simulink library "ttc"  (Simulink 8.2)
settings: Solver=ode45  StartTime=0.0  StopTime=10.0  RelTol=1e-3
undefined symbols (not defined in the file or in its folder): KIFO_OffsetToBumper_m
libraries: tcc x4, idiada_lib x1
settings Model: Creator=xsellart  LastModifiedBy=14069

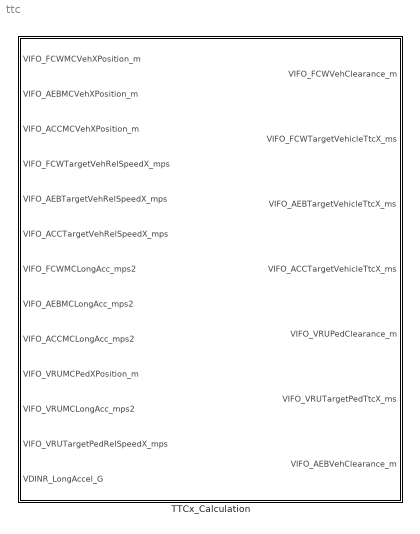
== system ttc ==
  TTCx_Calculation : Subsystem

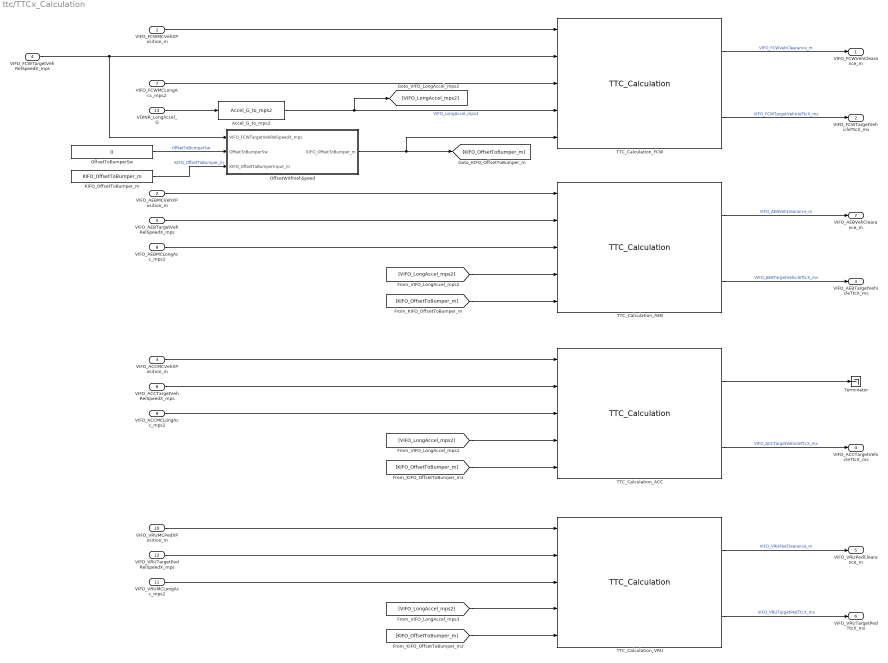
== system ttc/TTCx_Calculation ==
  VIFO_FCWMCVehXPosition_m : Inport
  VIFO_AEBMCVehXPosition_m : Inport  Port=2
  VIFO_ACCMCVehXPosition_m : Inport  Port=3
  VIFO_FCWTargetVehRelSpeedX_mps : Inport  Port=4
  VIFO_AEBTargetVehRelSpeedX_mps : Inport  Port=5
  VIFO_ACCTargetVehRelSpeedX_mps : Inport  Port=6
  VIFO_FCWMCLongAcc_mps2 : Inport  Port=7
  VIFO_AEBMCLongAcc_mps2 : Inport  Port=8
  VIFO_ACCMCLongAcc_mps2 : Inport  Port=9
  VIFO_VRUMCPedXPosition_m : Inport  Port=10
  VIFO_VRUMCLongAcc_mps2 : Inport  Port=11
  VIFO_VRUTargetPedRelSpeedX_mps : Inport  Port=12
  VDINR_LongAccel_G : Inport  Port=13
  Accel_G_to_mps2 : idiada_lib/Accel_G_to_mps2
  KIFO_OffsetToBumper_m : Constant  Value=KIFO_OffsetToBumper_m
  OffsetToBumperSw : Constant  Value=0
  OffsetWithVehSpeed : Subsystem
  TTC_Calculation_ACC : tcc/TTC_Calculation
  TTC_Calculation_AEB : tcc/TTC_Calculation
  TTC_Calculation_FCW : tcc/TTC_Calculation
  TTC_Calculation_VRU : tcc/TTC_Calculation
  Terminator : Terminator
  VIFO_FCWVehClearance_m : Outport
  VIFO_FCWTargetVehicleTtcX_ms : Outport  Port=2
  VIFO_AEBTargetVehicleTtcX_ms : Outport  Port=3
  VIFO_ACCTargetVehicleTtcX_ms : Outport  Port=4
  VIFO_VRUPedClearance_m : Outport  Port=5
  VIFO_VRUTargetPedTtcX_ms : Outport  Port=6
  VIFO_AEBVehClearance_m : Outport  Port=7
  wires:
  [KIFO_OffsetToBumper_m] -> TTC_Calculation_ACC/5
  TTC_Calculation_ACC/2 -> VIFO_ACCTargetVehicleTtcX_ms/1  "VIFO_ACCTargetVehicleTtcX_ms"
  VIFO_ACCMCLongAcc_mps2/1 -> TTC_Calculation_ACC/3
  VIFO_ACCTargetVehRelSpeedX_mps/1 -> TTC_Calculation_ACC/2
  VIFO_ACCMCVehXPosition_m/1 -> TTC_Calculation_ACC/1
  [VIFO_LongAccel_mps2] -> TTC_Calculation_ACC/4
  TTC_Calculation_ACC/1 -> Terminator/1
  [KIFO_OffsetToBumper_m] -> TTC_Calculation_AEB/5
  KIFO_OffsetToBumper_m/1 -> OffsetWithVehSpeed/3(KIFO_OffsetToBumperInput_m)  "KIFO_OffsetToBumper_m"
  TTC_Calculation_AEB/2 -> VIFO_AEBTargetVehicleTtcX_ms/1  "VIFO_AEBTargetVehicleTtcX_ms"
  VIFO_AEBMCLongAcc_mps2/1 -> TTC_Calculation_AEB/3
  VIFO_AEBTargetVehRelSpeedX_mps/1 -> TTC_Calculation_AEB/2
  VIFO_AEBMCVehXPosition_m/1 -> TTC_Calculation_AEB/1
  [VIFO_LongAccel_mps2] -> TTC_Calculation_AEB/4
  TTC_Calculation_AEB/1 -> VIFO_AEBVehClearance_m/1  "VIFO_AEBVehClearance_m"
  TTC_Calculation_FCW/2 -> VIFO_FCWTargetVehicleTtcX_ms/1  "VIFO_FCWTargetVehicleTtcX_ms"
  TTC_Calculation_FCW/1 -> VIFO_FCWVehClearance_m/1  "VIFO_FCWVehClearance_m"
  VIFO_FCWMCLongAcc_mps2/1 -> TTC_Calculation_FCW/3
  VIFO_FCWTargetVehRelSpeedX_mps/1 -> OffsetWithVehSpeed/1(VIFO_FCWTargetVehRelSpeedX_mps), TTC_Calculation_FCW/2
  VIFO_FCWMCVehXPosition_m/1 -> TTC_Calculation_FCW/1
  Accel_G_to_mps2/1 -> TTC_Calculation_FCW/4, [VIFO_LongAccel_mps2]  "VIFO_LongAccel_mps2"
  VDINR_LongAccel_G/1 -> Accel_G_to_mps2/1
  VIFO_VRUMCPedXPosition_m/1 -> TTC_Calculation_VRU/1
  VIFO_VRUTargetPedRelSpeedX_mps/1 -> TTC_Calculation_VRU/2
  VIFO_VRUMCLongAcc_mps2/1 -> TTC_Calculation_VRU/3
  [KIFO_OffsetToBumper_m] -> TTC_Calculation_VRU/5
  [VIFO_LongAccel_mps2] -> TTC_Calculation_VRU/4
  TTC_Calculation_VRU/2 -> VIFO_VRUTargetPedTtcX_ms/1  "VIFO_VRUTargetPedTtcX_ms"
  TTC_Calculation_VRU/1 -> VIFO_VRUPedClearance_m/1  "VIFO_VRUPedClearance_m"
  OffsetWithVehSpeed/1(KIFO_OffsetToBumper_m) -> TTC_Calculation_FCW/5, [KIFO_OffsetToBumper_m]
  OffsetToBumperSw/1 -> OffsetWithVehSpeed/2(OffsetToBumperSw)  "OffsetToBumperSw"

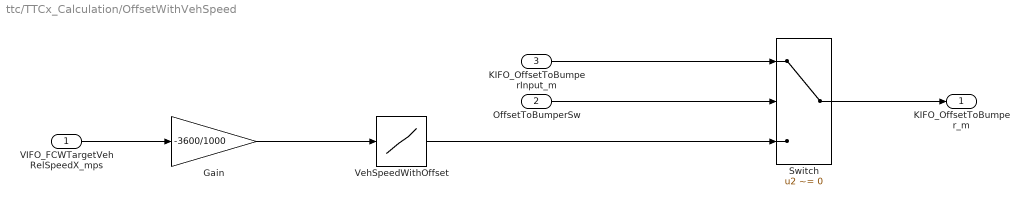
== system ttc/TTCx_Calculation/OffsetWithVehSpeed ==
  VIFO_FCWTargetVehRelSpeedX_mps : Inport
  OffsetToBumperSw : Inport  Port=2
  KIFO_OffsetToBumperInput_m : Inport  Port=3
  Gain : Gain  Gain=-3600/1000
  Switch : Switch  Criteria=u2 ~= 0
  VehSpeedWithOffset : Lookup  InputValues=[0 10 20 30 40 50 60 70]  Table=[0 0 0 0 -1 -1 -1 -1]  LookUpMeth=Interpolation-Use End Values
      settings: AttributesFormatString="Input=\"%<InputValues>\"\\nOutput=\"%<Table>\""
  KIFO_OffsetToBumper_m : Outport
  wires:
  VIFO_FCWTargetVehRelSpeedX_mps/1 -> Gain/1
  OffsetToBumperSw/1 -> Switch/2
  Switch/1 -> KIFO_OffsetToBumper_m/1
  KIFO_OffsetToBumperInput_m/1 -> Switch/1
  VehSpeedWithOffset/1 -> Switch/3
  Gain/1 -> VehSpeedWithOffset/1
